simulink model "SignalModelL7_hand"  (R2017a)
settings: Solver=FixedStepAuto  StartTime=0.0  StopTime=15  FixedStep=0.01  RelTol=1e-3
undefined symbols (not defined in the file): Ki, vKd, vKp
settings Model: Creator=roman  LastModifiedBy=roman

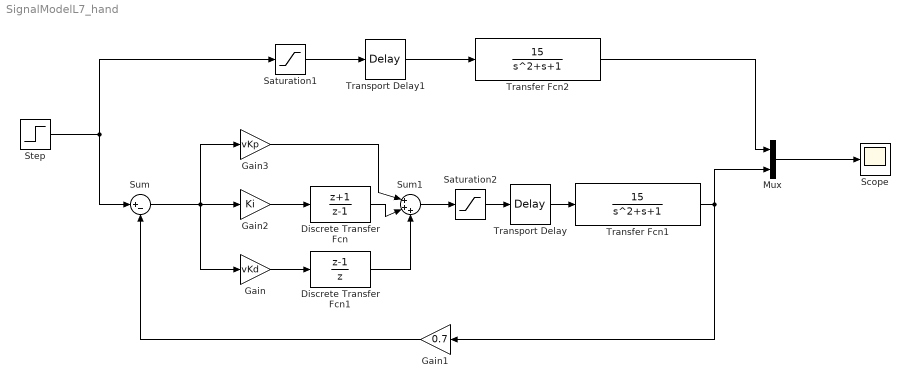
== system SignalModelL7_hand ==
  Discrete Transfer Fcn : DiscreteTransferFcn  Numerator=[1 1]  Denominator=[1 -1]  SampleTime=0.1
  Discrete Transfer Fcn1 : DiscreteTransferFcn  Numerator=[1 -1]  Denominator=[1 0]  SampleTime=0.1
  Gain : Gain  Gain=vKd
  Gain1 : Gain  Gain=0.7
  Gain2 : Gain  Gain=Ki
  Gain3 : Gain  Gain=vKp
  Mux : Mux  Inputs=2
  Saturation1 : Saturate  UpperLimit=200  LowerLimit=-200
  Saturation2 : Saturate  UpperLimit=200  LowerLimit=-200
  Scope : Scope
  Step : Step  Time=0  SampleTime=0
  Sum : Sum  Inputs=|+-
  Sum1 : Sum  Inputs=|+++
  Transfer Fcn1 : TransferFcn  Numerator=[15]  Denominator=[1 1 1]
  Transfer Fcn2 : TransferFcn  Numerator=[15]  Denominator=[1 1 1]
  Transport Delay : TransportDelay  DelayTime=0.1
  Transport Delay1 : TransportDelay  DelayTime=0.1
  wires:
  Transport Delay/1 -> Transfer Fcn1/1
  Transfer Fcn1/1 -> Mux/2, Gain1/1
  Transport Delay1/1 -> Transfer Fcn2/1
  Mux/1 -> Scope/1
  Saturation2/1 -> Transport Delay/1
  Sum/1 -> Gain3/1, Gain/1, Gain2/1
  Gain1/1 -> Sum/2
  Gain2/1 -> Discrete Transfer Fcn/1
  Sum1/1 -> Saturation2/1
  Saturation1/1 -> Transport Delay1/1
  Transfer Fcn2/1 -> Mux/1
  Step/1 -> Saturation1/1, Sum/1
  Gain/1 -> Discrete Transfer Fcn1/1
  Gain3/1 -> Sum1/1
  Discrete Transfer Fcn1/1 -> Sum1/3
  Discrete Transfer Fcn/1 -> Sum1/2
